simulink subsystem "V2VSimulator"  (R2024a)
settings: Solver=VariableStepAuto  StartTime=0.0  StopTime=10.0  RelTol=1e-3
undefined symbols (not defined in the file): SF_std, Ts
settings Model: Creator=The MathWorks, Inc.  LastModifiedBy=L03509110
settings SolverCC: MaxZcPerStep=1
settings OptimizationCC: ReuseModelBlockBuffer=off
settings ModelReferenceCC: EnableRefExpFcnMdlSchedulingChecks=on
settings RTWCC: GPUComputeCapability=3.5  DLArmComputeVersion=19.05

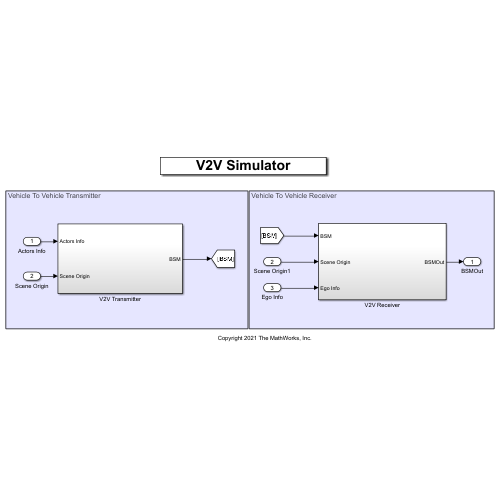
[thumbnail: Simulink's stored preview of the top-level diagram]
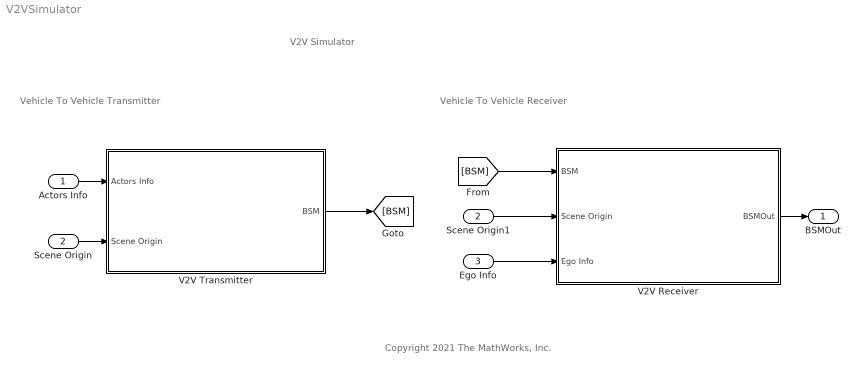
== system V2VSimulator ==
  note: Vehicle To Vehicle Transmitter
  note: V2V Simulator
  note: Vehicle To Vehicle Receiver
  note: Copyright 2021 The MathWorks, Inc.
  Actors Info : Inport
  Scene Origin : Inport  Port=2
  Ego Info : Inport  Port=3
  Scene Origin1 : InportShadow  Port=2
  V2V Receiver : Subsystem
  V2V Transmitter : Subsystem
  BSMOut : Outport
  wires:
  V2V Transmitter/1(BSM) -> [BSM]
  Actors Info/1 -> V2V Transmitter/1(Actors Info)
  Scene Origin/1 -> V2V Transmitter/2(Scene Origin)
  V2V Receiver/1(BSMOut) -> BSMOut/1
  [BSM] -> V2V Receiver/1(BSM)
  Ego Info/1 -> V2V Receiver/3(Ego Info)
  Scene Origin1/1 -> V2V Receiver/2(Scene Origin)

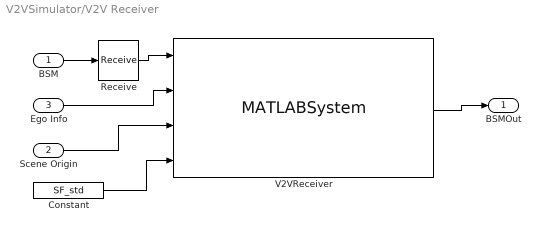
== system V2VSimulator/V2V Receiver ==
  BSM : Inport  OutDataTypeStr=Bus: BusBSM  BusOutputAsStruct=on
  Scene Origin : Inport  Port=2  PortDimensions=[1 3]  BusOutputAsStruct=on
  Ego Info : Inport  Port=3  OutDataTypeStr=Bus: BusVehiclePose  BusOutputAsStruct=on
  Constant : Constant  Value=SF_std
  Receive : Receive  InputPortMessageModes=m  UseInternalQueue=off  QueueOverwriting=on  QueueLength=1  QueueType=LIFO
  V2VReceiver : MATLABSystem  System=HelperV2VReceiver  SnrCurves=channelAttributes  OutputStruct=Simulink.Bus.createMATLABStruct('BusBSM')  SimulateUsing=Code generation
      mask Type: HelperV2VReceiver
      mask Display:
      | disp('HelperV2VReceiver');
      | port_label('input',1,'bsm');
      | port_label('input',2,'egoPose');
      | port_label('input',3,'sceneOrigin');
      | port_label('input',4,'SF_std');
      | port_label('output',1,'bsmOut');
  BSMOut : Outport  OutDataTypeStr=Bus: BusBSM  BusOutputAsStruct=on
  wires:
  Constant/1 -> V2VReceiver/4
  Ego Info/1 -> V2VReceiver/2
  Receive/1 -> V2VReceiver/1
  V2VReceiver/1 -> BSMOut/1
  Scene Origin/1 -> V2VReceiver/3
  BSM/1 -> Receive/1

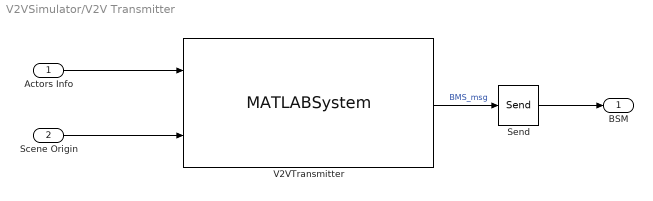
== system V2VSimulator/V2V Transmitter ==
  Actors Info : Inport  OutDataTypeStr=Bus: BusActorsInfo  BusOutputAsStruct=on
  Scene Origin : Inport  Port=2  PortDimensions=[1 3]
  Send : Send  OutputPortMessageModes=m
  V2VTransmitter : MATLABSystem  System=HelperV2VTransmitter  SampleTime=Ts  OutputStruct=Simulink.Bus.createMATLABStruct('BusBSM')  SimulateUsing=Code generation
      mask Type: HelperV2VTransmitter
      mask Display:
      | disp('HelperV2VTransmitter');
      | port_label('input',1,'actorsInfo');
      | port_label('input',2,'sceneOrigin');
      | port_label('output',1,'bsm');
  BSM : Outport  OutDataTypeStr=Bus: BusBSM  BusOutputAsStruct=on
  wires:
  Send/1 -> BSM/1
  V2VTransmitter/1 -> Send/1  "BMS_msg"
  Scene Origin/1 -> V2VTransmitter/2
  Actors Info/1 -> V2VTransmitter/1
